simulink model "Compare"  (R2016b)
settings: Solver=VariableStepAuto  StartTime=0.0  StopTime=10.0  RelTol=1e-3
settings Model: Creator=user  LastModifiedBy=user

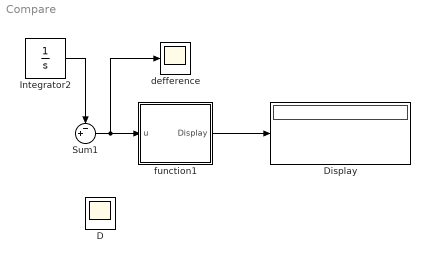
== system Compare ==
  D : Scope
  Display : Display
  Integrator2 : Integrator  InitialConditionSource=external
  Sum1 : Sum  Inputs=-+|
  defference : Scope
  function1 : Subsystem
  wires:
  function1/1(Display) -> Display/1
  Sum1/1 -> defference/1, function1/1(u)
  ? -> Integrator2/2, Sum1/2, D/1
  ? -> Integrator2/1
  Integrator2/1 -> Sum1/1

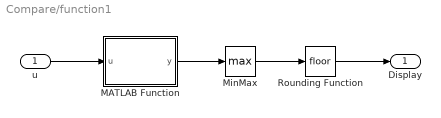
== system Compare/function1 ==
  u : Inport
  MATLAB Function : MATLAB Function  TreatAsAtomicUnit=on
  MinMax : MinMax  Function=max  OutMin=1e-16
  Rounding Function : Rounding
  Display : Outport
  wires:
  MATLAB Function/1(y) -> MinMax/1
  MinMax/1 -> Rounding Function/1
  u/1 -> MATLAB Function/1(u)
  Rounding Function/1 -> Display/1

== matlab function Compare/function1/MATLAB Function ==
  data: u input; y output
function y = fcn(u)
%#codegen
persistent initial_value

if(isempty(initial_value))
    initial_value = u;
end

y = log10(abs((u-initial_value)));
